simulink model "CMOS_Kernel_Memory_Sync"  (R2023b)
settings: Solver=VariableStepAuto  StartTime=0.0  StopTime=30000000  RelTol=1e-3
values from neighbouring files (symbols this model uses):
  AmountOfPixelsPerScanline = 400    [Kernel_Setup_Script.m]
  AmountOfRamBlocksScanlines = 5    [Kernel_Setup_Script.m]
  AmountOfRamBlocksScanlinesOffset = AmountOfRamBlocksScanlines - 1    (= 4)    [Kernel_Setup_Script.m]
  AmountOfScanlinePixels = 73700    [Kernel_Setup_Script.m]
  AmountOfScanlinePixelsOffset = AmountOfScanlinePixels - 1    (= 73699)    [Kernel_Setup_Script.m]
  AmountOfScanlines = 1100    [Kernel_Setup_Script.m]
  AmountOfScanlinesOffset = AmountOfScanlines - 1    (= 1099)    [Kernel_Setup_Script.m]
  AOPPK_Off = AmountOfPixelsPerScanline - 1    (= 399)    [Kernel_Setup_Script.m]
  AOPPS_Off = AmountOfPixelsPerScanline - 1    (= 399)    [Kernel_Setup_Script.m]
  FramePackOff_0 = FramePackOff_0 - ScanlineFifoCheck    [Kernel_Setup_Script.m]
  FramePackOff_1 = FramePackOff_1 - ScanlineFifoCheck    [Kernel_Setup_Script.m]
  FramePackOff_2 = FramePackOff_2 - ScanlineFifoCheck    [Kernel_Setup_Script.m]
  FramePackOff_3 = FramePackOff_3 - ScanlineFifoCheck    [Kernel_Setup_Script.m]
  FramePackOff_4 = FramePackOff_4 - ScanlineFifoCheck    [Kernel_Setup_Script.m]
  FramePackOff_5 = FramePackOff_5 - ScanlineFifoCheck    [Kernel_Setup_Script.m]
  KernelPackOff_0 = KernelPackOff_0 - KernelBitsPerRow    [Kernel_Setup_Script.m]
  KernelPackOff_1 = KernelPackOff_1 - KernelBitsPerRow    [Kernel_Setup_Script.m]
  KernelPackOff_2 = KernelPackOff_2 - KernelBitsPerRow    [Kernel_Setup_Script.m]
  KernelPackOff_3 = KernelPackOff_3 - KernelBitsPerRow    [Kernel_Setup_Script.m]
  Slice59DownTo48Top = (MsbOffset - (ScanlinePixelBitSizeController*1))    (= 59)    [Kernel_Setup_Script.m]
  Slice71DownTo60Top = (MsbOffset - (ScanlinePixelBitSizeController*0))    (= 71)    [Kernel_Setup_Script.m]
  TotalSectionsForFrames = AmountOfScanlines/AmountOfRamBlocksScanlines    (= 220)    [Kernel_Setup_Script.m]
  UltraRamRows = AmountOfPixelsPerScanline/ScanlineFifoCheck    [Kernel_Setup_Script.m]
  UltraRamRowsCeil = ceil(AmountOfPixelsPerScanline/ScanlineFifoCheck)    [Kernel_Setup_Script.m]
  UltraRamRowsKernel = AmountOfPixelsPerScanline/KernelBitsPerRow    (= 100)    [Kernel_Setup_Script.m]
  UltraRamRowsKernelCeil = ceil(AmountOfPixelsPerScanline/KernelBitsPerRow)    [Kernel_Setup_Script.m]
  UltraRamRowsMemorySectionOffset = UltraRamRowsCeil*AmountOfRamBlocksScanlines    [Kernel_Setup_Script.m]
  UltraRamRowsOffset = UltraRamRowsCeil - 1    [Kernel_Setup_Script.m]
undefined symbols (not defined in the file or in its folder): c, Down, sfvc784, Up, xck26
libraries: hdlBasic x4512, vmcUtilities x1
(part 35 of 39)

== system CMOS_Kernel_Memory_Sync/Memory Handler/Math/Kernel Result 9/Accumulator Offset 0 ==
  Input Value : Inport
  Input Valid : Inport  Port=2
  Last Row : Inport  Port=3
  Hard Reset : Inport  Port=4
  Accumulator 0 : hdlBasic/Accumulator  operation=Add  n_bits=64  overflow=Wrap  scale=1  rst=on  hasbypass=off  en=off  latency=1  msb_inp=100  msb=100  lsb=-100  use_behavioral_HDL=on  implementation=Fabric  XmcBlockStatus=1  maskContainerNames=group3  block_type=accum  block_config=sysgen:Accum_config  block_width=566  block_height=845
  Constant : hdlBasic/Constant  const=0  gui_display_data_type=Fixed-point  arith_type=Unsigned  n_bits=18  bin_pt=0  preci_type=Single  exp_width=8  frac_width=24  explicit_period=off  period=1  XmcBlockStatus=1  maskContainerNames=tabcontainer1  block_type=constant  block_config=sysgen:Constant_config
  Delay1 : hdlBasic/Delay  rst=off  en=off  latency=1  reg_retiming=off  XmcBlockStatus=1  maskContainerNames=group1  block_type=delay  block_config=sysgen:Delay_config
  Delay2 : hdlBasic/Delay  rst=off  en=off  latency=1  reg_retiming=off  XmcBlockStatus=1  maskContainerNames=group1  block_type=delay  block_config=sysgen:Delay_config
  Logical : hdlBasic/Logical  logical_function=AND  inputs=2  en=off  latency=1  precision=Full  arith_type=Unsigned  n_bits=16  bin_pt=0  align_bp=on  overflow=[]  quantization=[]  XmcBlockStatus=1  maskContainerNames=tabcontainer1  block_type=logical  block_config=sysgen:Logical_config
  Logical1 : hdlBasic/Logical  logical_function=OR  inputs=2  en=off  latency=1  precision=Full  arith_type=Unsigned  n_bits=16  bin_pt=0  align_bp=on  overflow=[]  quantization=[]  XmcBlockStatus=1  maskContainerNames=tabcontainer1  block_type=logical  block_config=sysgen:Logical_config
  Mux : hdlBasic/Mux  inputs=2  en=off  latency=1  precision=Full  arith_type=Unsigned  n_bits=16  bin_pt=14  quantization=Truncate  overflow=Wrap  XmcBlockStatus=1  maskContainerNames=tabcontainer1  block_type=mux  block_config=sysgen:Mux_config
  Accumulator Output : Outport
  Accumulator Valid : Outport  Port=2
  wires:
  Accumulator 0/1 -> Accumulator Output/1
  Input Valid/1 -> Logical/1, Mux/1
  Input Value/1 -> Mux/3
  Mux/1 -> Accumulator 0/1
  Last Row/1 -> Logical/2
  Constant/1 -> Mux/2
  Delay1/1 -> Accumulator 0/2
  Logical/1 -> Logical1/2, Delay2/1
  Delay2/1 -> Accumulator Valid/1
  Logical1/1 -> Delay1/1
  Hard Reset/1 -> Logical1/1

== system CMOS_Kernel_Memory_Sync/Memory Handler/Math/Kernel Result 9/Accumulator Offset 1 ==
  Input Value : Inport
  Input Valid : Inport  Port=2
  Last Row : Inport  Port=3
  Hard Reset : Inport  Port=4
  Accumulator 0 : hdlBasic/Accumulator  operation=Add  n_bits=64  overflow=Wrap  scale=1  rst=on  hasbypass=off  en=off  latency=1  msb_inp=100  msb=100  lsb=-100  use_behavioral_HDL=on  implementation=Fabric  XmcBlockStatus=1  maskContainerNames=group3  block_type=accum  block_config=sysgen:Accum_config  block_width=566  block_height=845
  Constant : hdlBasic/Constant  const=0  gui_display_data_type=Fixed-point  arith_type=Unsigned  n_bits=18  bin_pt=0  preci_type=Single  exp_width=8  frac_width=24  explicit_period=off  period=1  XmcBlockStatus=1  maskContainerNames=tabcontainer1  block_type=constant  block_config=sysgen:Constant_config
  Delay1 : hdlBasic/Delay  rst=off  en=off  latency=1  reg_retiming=off  XmcBlockStatus=1  maskContainerNames=group1  block_type=delay  block_config=sysgen:Delay_config
  Delay2 : hdlBasic/Delay  rst=off  en=off  latency=1  reg_retiming=off  XmcBlockStatus=1  maskContainerNames=group1  block_type=delay  block_config=sysgen:Delay_config
  Logical : hdlBasic/Logical  logical_function=AND  inputs=2  en=off  latency=1  precision=Full  arith_type=Unsigned  n_bits=16  bin_pt=0  align_bp=on  overflow=[]  quantization=[]  XmcBlockStatus=1  maskContainerNames=tabcontainer1  block_type=logical  block_config=sysgen:Logical_config
  Logical1 : hdlBasic/Logical  logical_function=OR  inputs=2  en=off  latency=1  precision=Full  arith_type=Unsigned  n_bits=16  bin_pt=0  align_bp=on  overflow=[]  quantization=[]  XmcBlockStatus=1  maskContainerNames=tabcontainer1  block_type=logical  block_config=sysgen:Logical_config
  Mux : hdlBasic/Mux  inputs=2  en=off  latency=1  precision=Full  arith_type=Unsigned  n_bits=16  bin_pt=14  quantization=Truncate  overflow=Wrap  XmcBlockStatus=1  maskContainerNames=tabcontainer1  block_type=mux  block_config=sysgen:Mux_config
  Accumulator Output : Outport
  Accumulator Valid : Outport  Port=2
  wires:
  Accumulator 0/1 -> Accumulator Output/1
  Input Valid/1 -> Logical/1, Mux/1
  Input Value/1 -> Mux/3
  Mux/1 -> Accumulator 0/1
  Last Row/1 -> Logical/2
  Constant/1 -> Mux/2
  Delay1/1 -> Accumulator 0/2
  Logical/1 -> Logical1/2, Delay2/1
  Delay2/1 -> Accumulator Valid/1
  Logical1/1 -> Delay1/1
  Hard Reset/1 -> Logical1/1

== system CMOS_Kernel_Memory_Sync/Memory Handler/Math/Kernel Result 9/Accumulator Offset 2 ==
  Input Value : Inport
  Input Valid : Inport  Port=2
  Last Row : Inport  Port=3
  Hard Reset : Inport  Port=4
  Accumulator 0 : hdlBasic/Accumulator  operation=Add  n_bits=64  overflow=Wrap  scale=1  rst=on  hasbypass=off  en=off  latency=1  msb_inp=100  msb=100  lsb=-100  use_behavioral_HDL=on  implementation=Fabric  XmcBlockStatus=1  maskContainerNames=group3  block_type=accum  block_config=sysgen:Accum_config  block_width=566  block_height=845
  Constant : hdlBasic/Constant  const=0  gui_display_data_type=Fixed-point  arith_type=Unsigned  n_bits=18  bin_pt=0  preci_type=Single  exp_width=8  frac_width=24  explicit_period=off  period=1  XmcBlockStatus=1  maskContainerNames=tabcontainer1  block_type=constant  block_config=sysgen:Constant_config
  Delay1 : hdlBasic/Delay  rst=off  en=off  latency=1  reg_retiming=off  XmcBlockStatus=1  maskContainerNames=group1  block_type=delay  block_config=sysgen:Delay_config
  Delay2 : hdlBasic/Delay  rst=off  en=off  latency=1  reg_retiming=off  XmcBlockStatus=1  maskContainerNames=group1  block_type=delay  block_config=sysgen:Delay_config
  Logical : hdlBasic/Logical  logical_function=AND  inputs=2  en=off  latency=1  precision=Full  arith_type=Unsigned  n_bits=16  bin_pt=0  align_bp=on  overflow=[]  quantization=[]  XmcBlockStatus=1  maskContainerNames=tabcontainer1  block_type=logical  block_config=sysgen:Logical_config
  Logical1 : hdlBasic/Logical  logical_function=OR  inputs=2  en=off  latency=1  precision=Full  arith_type=Unsigned  n_bits=16  bin_pt=0  align_bp=on  overflow=[]  quantization=[]  XmcBlockStatus=1  maskContainerNames=tabcontainer1  block_type=logical  block_config=sysgen:Logical_config
  Mux : hdlBasic/Mux  inputs=2  en=off  latency=1  precision=Full  arith_type=Unsigned  n_bits=16  bin_pt=14  quantization=Truncate  overflow=Wrap  XmcBlockStatus=1  maskContainerNames=tabcontainer1  block_type=mux  block_config=sysgen:Mux_config
  Accumulator Output : Outport
  Accumulator Valid : Outport  Port=2
  wires:
  Accumulator 0/1 -> Accumulator Output/1
  Input Valid/1 -> Logical/1, Mux/1
  Input Value/1 -> Mux/3
  Mux/1 -> Accumulator 0/1
  Last Row/1 -> Logical/2
  Constant/1 -> Mux/2
  Delay1/1 -> Accumulator 0/2
  Logical/1 -> Logical1/2, Delay2/1
  Delay2/1 -> Accumulator Valid/1
  Logical1/1 -> Delay1/1
  Hard Reset/1 -> Logical1/1

== system CMOS_Kernel_Memory_Sync/Memory Handler/Math/Kernel Result 9/Accumulator Offset 3 ==
  Input Value : Inport
  Input Valid : Inport  Port=2
  Last Row : Inport  Port=3
  Hard Reset : Inport  Port=4
  Accumulator 0 : hdlBasic/Accumulator  operation=Add  n_bits=64  overflow=Wrap  scale=1  rst=on  hasbypass=off  en=off  latency=1  msb_inp=100  msb=100  lsb=-100  use_behavioral_HDL=on  implementation=Fabric  XmcBlockStatus=1  maskContainerNames=group3  block_type=accum  block_config=sysgen:Accum_config  block_width=566  block_height=845
  Constant : hdlBasic/Constant  const=0  gui_display_data_type=Fixed-point  arith_type=Unsigned  n_bits=18  bin_pt=0  preci_type=Single  exp_width=8  frac_width=24  explicit_period=off  period=1  XmcBlockStatus=1  maskContainerNames=tabcontainer1  block_type=constant  block_config=sysgen:Constant_config
  Delay1 : hdlBasic/Delay  rst=off  en=off  latency=1  reg_retiming=off  XmcBlockStatus=1  maskContainerNames=group1  block_type=delay  block_config=sysgen:Delay_config
  Delay2 : hdlBasic/Delay  rst=off  en=off  latency=1  reg_retiming=off  XmcBlockStatus=1  maskContainerNames=group1  block_type=delay  block_config=sysgen:Delay_config
  Logical : hdlBasic/Logical  logical_function=AND  inputs=2  en=off  latency=1  precision=Full  arith_type=Unsigned  n_bits=16  bin_pt=0  align_bp=on  overflow=[]  quantization=[]  XmcBlockStatus=1  maskContainerNames=tabcontainer1  block_type=logical  block_config=sysgen:Logical_config
  Logical1 : hdlBasic/Logical  logical_function=OR  inputs=2  en=off  latency=1  precision=Full  arith_type=Unsigned  n_bits=16  bin_pt=0  align_bp=on  overflow=[]  quantization=[]  XmcBlockStatus=1  maskContainerNames=tabcontainer1  block_type=logical  block_config=sysgen:Logical_config
  Mux : hdlBasic/Mux  inputs=2  en=off  latency=1  precision=Full  arith_type=Unsigned  n_bits=16  bin_pt=14  quantization=Truncate  overflow=Wrap  XmcBlockStatus=1  maskContainerNames=tabcontainer1  block_type=mux  block_config=sysgen:Mux_config
  Accumulator Output : Outport
  Accumulator Valid : Outport  Port=2
  wires:
  Accumulator 0/1 -> Accumulator Output/1
  Input Valid/1 -> Logical/1, Mux/1
  Input Value/1 -> Mux/3
  Mux/1 -> Accumulator 0/1
  Last Row/1 -> Logical/2
  Constant/1 -> Mux/2
  Delay1/1 -> Accumulator 0/2
  Logical/1 -> Logical1/2, Delay2/1
  Delay2/1 -> Accumulator Valid/1
  Logical1/1 -> Delay1/1
  Hard Reset/1 -> Logical1/1

== system CMOS_Kernel_Memory_Sync/Memory Handler/Math/Kernel Result 9/Accumulator Offset 4 ==
  Input Value : Inport
  Input Valid : Inport  Port=2
  Last Row : Inport  Port=3
  Hard Reset : Inport  Port=4
  Accumulator 0 : hdlBasic/Accumulator  operation=Add  n_bits=64  overflow=Wrap  scale=1  rst=on  hasbypass=off  en=off  latency=1  msb_inp=100  msb=100  lsb=-100  use_behavioral_HDL=on  implementation=Fabric  XmcBlockStatus=1  maskContainerNames=group3  block_type=accum  block_config=sysgen:Accum_config  block_width=566  block_height=845
  Constant : hdlBasic/Constant  const=0  gui_display_data_type=Fixed-point  arith_type=Unsigned  n_bits=18  bin_pt=0  preci_type=Single  exp_width=8  frac_width=24  explicit_period=off  period=1  XmcBlockStatus=1  maskContainerNames=tabcontainer1  block_type=constant  block_config=sysgen:Constant_config
  Delay1 : hdlBasic/Delay  rst=off  en=off  latency=1  reg_retiming=off  XmcBlockStatus=1  maskContainerNames=group1  block_type=delay  block_config=sysgen:Delay_config
  Delay2 : hdlBasic/Delay  rst=off  en=off  latency=1  reg_retiming=off  XmcBlockStatus=1  maskContainerNames=group1  block_type=delay  block_config=sysgen:Delay_config
  Logical : hdlBasic/Logical  logical_function=AND  inputs=2  en=off  latency=1  precision=Full  arith_type=Unsigned  n_bits=16  bin_pt=0  align_bp=on  overflow=[]  quantization=[]  XmcBlockStatus=1  maskContainerNames=tabcontainer1  block_type=logical  block_config=sysgen:Logical_config
  Logical1 : hdlBasic/Logical  logical_function=OR  inputs=2  en=off  latency=1  precision=Full  arith_type=Unsigned  n_bits=16  bin_pt=0  align_bp=on  overflow=[]  quantization=[]  XmcBlockStatus=1  maskContainerNames=tabcontainer1  block_type=logical  block_config=sysgen:Logical_config
  Mux : hdlBasic/Mux  inputs=2  en=off  latency=1  precision=Full  arith_type=Unsigned  n_bits=16  bin_pt=14  quantization=Truncate  overflow=Wrap  XmcBlockStatus=1  maskContainerNames=tabcontainer1  block_type=mux  block_config=sysgen:Mux_config
  Accumulator Output : Outport
  Accumulator Valid : Outport  Port=2
  wires:
  Accumulator 0/1 -> Accumulator Output/1
  Input Valid/1 -> Logical/1, Mux/1
  Input Value/1 -> Mux/3
  Mux/1 -> Accumulator 0/1
  Last Row/1 -> Logical/2
  Constant/1 -> Mux/2
  Delay1/1 -> Accumulator 0/2
  Logical/1 -> Logical1/2, Delay2/1
  Delay2/1 -> Accumulator Valid/1
  Logical1/1 -> Delay1/1
  Hard Reset/1 -> Logical1/1

== system CMOS_Kernel_Memory_Sync/Memory Handler/Math/Kernel Result 9/Multiple and Add Offset 0 ==
  Pixel 0 : Inport
  Weight 0 : Inport  Port=2
  Pixel 1 : Inport  Port=3
  Weight 1 : Inport  Port=4
  Pixel 2 : Inport  Port=5
  Weight 2 : Inport  Port=6
  Pixel 3 : Inport  Port=7
  Weight 3 : Inport  Port=8
  Pixel 4 : Inport  Port=9
  Weight 4 : Inport  Port=10
  Pixel 5 : Inport  Port=11
  Weight 5 : Inport  Port=12
  Pixel 6 : Inport  Port=13
  Weight 6 : Inport  Port=14
  Pixel 7 : Inport  Port=15
  Weight 7 : Inport  Port=16
  Pixel 8 : Inport  Port=17
  Weight 8 : Inport  Port=18
  Pixel 9 : Inport  Port=19
  Weight 9 : Inport  Port=20
  Pixel 10 : Inport  Port=21
  Weight 10 : Inport  Port=22
  Pixel 11 : Inport  Port=23
  Weight 11 : Inport  Port=24
  Valid Data : Inport  Port=25
  "Combine ((0-1)-(2-3)) - ((4-5)-(6-7)) " : hdlBasic/AddSub  mode=Addition  use_carryin=off  use_carryout=off  en=off  latency=1  precision=Full  arith_type=Unsigned  n_bits=21  bin_pt=0  quantization=Truncate  overflow=Wrap  use_behavioral_HDL=off  hw_selection=Fabric  pipelined=off  XmcBlockStatus=1  maskContainerNames=tabcontainer1  block_type=addsub  block_config=sysgen:Addsub_config
  Combine (0-1)-(2-3) : hdlBasic/AddSub  mode=Addition  use_carryin=off  use_carryout=off  en=off  latency=1  precision=Full  arith_type=Unsigned  n_bits=20  bin_pt=0  quantization=Truncate  overflow=Wrap  use_behavioral_HDL=off  hw_selection=Fabric  pipelined=off  XmcBlockStatus=1  maskContainerNames=tabcontainer1  block_type=addsub  block_config=sysgen:Addsub_config
  Combine (4-5)-(6-7) : hdlBasic/AddSub  mode=Addition  use_carryin=off  use_carryout=off  en=off  latency=1  precision=Full  arith_type=Unsigned  n_bits=20  bin_pt=0  quantization=Truncate  overflow=Wrap  use_behavioral_HDL=off  hw_selection=Fabric  pipelined=off  XmcBlockStatus=1  maskContainerNames=tabcontainer1  block_type=addsub  block_config=sysgen:Addsub_config
  Combine (8-9)-(10-11) : hdlBasic/AddSub  mode=Addition  use_carryin=off  use_carryout=off  en=off  latency=1  precision=Full  arith_type=Unsigned  n_bits=20  bin_pt=0  quantization=Truncate  overflow=Wrap  use_behavioral_HDL=off  hw_selection=Fabric  pipelined=off  XmcBlockStatus=1  maskContainerNames=tabcontainer1  block_type=addsub  block_config=sysgen:Addsub_config
  Combine 0-1 : hdlBasic/AddSub  mode=Addition  use_carryin=off  use_carryout=off  en=off  latency=1  precision=Full  arith_type=Unsigned  n_bits=31  bin_pt=0  quantization=Truncate  overflow=Wrap  use_behavioral_HDL=off  hw_selection=Fabric  pipelined=off  XmcBlockStatus=1  maskContainerNames=tabcontainer1  block_type=addsub  block_config=sysgen:Addsub_config
  Combine 10-11 : hdlBasic/AddSub  mode=Addition  use_carryin=off  use_carryout=off  en=off  latency=1  precision=Full  arith_type=Unsigned  n_bits=19  bin_pt=0  quantization=Truncate  overflow=Wrap  use_behavioral_HDL=off  hw_selection=Fabric  pipelined=off  XmcBlockStatus=1  maskContainerNames=tabcontainer1  block_type=addsub  block_config=sysgen:Addsub_config
  Combine 2-3 : hdlBasic/AddSub  mode=Addition  use_carryin=off  use_carryout=off  en=off  latency=1  precision=Full  arith_type=Unsigned  n_bits=19  bin_pt=0  quantization=Truncate  overflow=Wrap  use_behavioral_HDL=off  hw_selection=Fabric  pipelined=off  XmcBlockStatus=1  maskContainerNames=tabcontainer1  block_type=addsub  block_config=sysgen:Addsub_config
  Combine 4-5 : hdlBasic/AddSub  mode=Addition  use_carryin=off  use_carryout=off  en=off  latency=1  precision=Full  arith_type=Unsigned  n_bits=19  bin_pt=0  quantization=Truncate  overflow=Wrap  use_behavioral_HDL=off  hw_selection=Fabric  pipelined=off  XmcBlockStatus=1  maskContainerNames=tabcontainer1  block_type=addsub  block_config=sysgen:Addsub_config
  Combine 6-7 : hdlBasic/AddSub  mode=Addition  use_carryin=off  use_carryout=off  en=off  latency=1  precision=Full  arith_type=Unsigned  n_bits=19  bin_pt=0  quantization=Truncate  overflow=Wrap  use_behavioral_HDL=off  hw_selection=Fabric  pipelined=off  XmcBlockStatus=1  maskContainerNames=tabcontainer1  block_type=addsub  block_config=sysgen:Addsub_config
  Combine 8-9 : hdlBasic/AddSub  mode=Addition  use_carryin=off  use_carryout=off  en=off  latency=1  precision=Full  arith_type=Unsigned  n_bits=19  bin_pt=0  quantization=Truncate  overflow=Wrap  use_behavioral_HDL=off  hw_selection=Fabric  pipelined=off  XmcBlockStatus=1  maskContainerNames=tabcontainer1  block_type=addsub  block_config=sysgen:Addsub_config
  Delay Addition{,2..4} (4 alike) : hdlBasic/Delay  rst=off  en=off  latency=1  reg_retiming=off  XmcBlockStatus=1  maskContainerNames=group1  block_type=delay  block_config=sysgen:Delay_config
  Delay Addition 2 : hdlBasic/Delay  rst=off  en=off  latency=1  reg_retiming=off  XmcBlockStatus=1  maskContainerNames=group1  block_type=delay  block_config=sysgen:Delay_config
  Delay Addition1 : hdlBasic/Delay  rst=off  en=off  latency=3  reg_retiming=off  XmcBlockStatus=1  maskContainerNames=group1  block_type=delay  block_config=sysgen:Delay_config
  Last Combine : hdlBasic/AddSub  mode=Addition  use_carryin=off  use_carryout=off  en=off  latency=1  precision=Full  arith_type=Unsigned  n_bits=22  bin_pt=0  quantization=Truncate  overflow=Wrap  use_behavioral_HDL=off  hw_selection=Fabric  pipelined=off  XmcBlockStatus=1  maskContainerNames=tabcontainer1  block_type=addsub  block_config=sysgen:Addsub_config
  Pixel 0 X Weight 0 : hdlBasic/Mult  precision=User Defined  arith_type=Unsigned  n_bits=30  bin_pt=0  quantization=Truncate  overflow=Wrap  en=off  latency=3  use_behavioral_HDL=off  opt=Speed  use_embedded=on  optimum_pipeline=off  pipeline=on  use_rpm=on  placement_style=Triangular  XmcBlockStatus=1  maskContainerNames=group1  block_type=mult  block_config=sysgen:Mult_config  block_width=598  block_height=876
  Pixel 1 X Weight 1 : hdlBasic/Mult  precision=User Defined  arith_type=Unsigned  n_bits=30  bin_pt=0  quantization=Truncate  overflow=Wrap  en=off  latency=3  use_behavioral_HDL=off  opt=Speed  use_embedded=on  optimum_pipeline=off  pipeline=on  use_rpm=on  placement_style=Triangular  XmcBlockStatus=1  maskContainerNames=group1  block_type=mult  block_config=sysgen:Mult_config  block_width=598  block_height=876
  Pixel 10 X Weight 10 : hdlBasic/Mult  precision=User Defined  arith_type=Unsigned  n_bits=30  bin_pt=0  quantization=Truncate  overflow=Wrap  en=off  latency=3  use_behavioral_HDL=off  opt=Speed  use_embedded=on  optimum_pipeline=off  pipeline=on  use_rpm=on  placement_style=Triangular  XmcBlockStatus=1  maskContainerNames=group1  block_type=mult  block_config=sysgen:Mult_config  block_width=598  block_height=876
  Pixel 11 X Weight 11 : hdlBasic/Mult  precision=User Defined  arith_type=Unsigned  n_bits=30  bin_pt=0  quantization=Truncate  overflow=Wrap  en=off  latency=3  use_behavioral_HDL=off  opt=Speed  use_embedded=on  optimum_pipeline=off  pipeline=on  use_rpm=on  placement_style=Triangular  XmcBlockStatus=1  maskContainerNames=group1  block_type=mult  block_config=sysgen:Mult_config  block_width=598  block_height=876
  Pixel 2 X Weight 2 : hdlBasic/Mult  precision=User Defined  arith_type=Unsigned  n_bits=30  bin_pt=0  quantization=Truncate  overflow=Wrap  en=off  latency=3  use_behavioral_HDL=off  opt=Speed  use_embedded=on  optimum_pipeline=off  pipeline=on  use_rpm=on  placement_style=Triangular  XmcBlockStatus=1  maskContainerNames=group1  block_type=mult  block_config=sysgen:Mult_config  block_width=598  block_height=876
  Pixel 3 X Weight 3 : hdlBasic/Mult  precision=User Defined  arith_type=Unsigned  n_bits=30  bin_pt=0  quantization=Truncate  overflow=Wrap  en=off  latency=3  use_behavioral_HDL=off  opt=Speed  use_embedded=on  optimum_pipeline=off  pipeline=on  use_rpm=on  placement_style=Triangular  XmcBlockStatus=1  maskContainerNames=group1  block_type=mult  block_config=sysgen:Mult_config  block_width=598  block_height=876
  Pixel 4 X Weight 4 : hdlBasic/Mult  precision=User Defined  arith_type=Unsigned  n_bits=30  bin_pt=0  quantization=Truncate  overflow=Wrap  en=off  latency=3  use_behavioral_HDL=off  opt=Speed  use_embedded=on  optimum_pipeline=off  pipeline=on  use_rpm=on  placement_style=Triangular  XmcBlockStatus=1  maskContainerNames=group1  block_type=mult  block_config=sysgen:Mult_config  block_width=598  block_height=876
  Pixel 5 X Weight 5 : hdlBasic/Mult  precision=User Defined  arith_type=Unsigned  n_bits=30  bin_pt=0  quantization=Truncate  overflow=Wrap  en=off  latency=3  use_behavioral_HDL=off  opt=Speed  use_embedded=on  optimum_pipeline=off  pipeline=on  use_rpm=on  placement_style=Triangular  XmcBlockStatus=1  maskContainerNames=group1  block_type=mult  block_config=sysgen:Mult_config  block_width=598  block_height=876
  Pixel 6 X Weight 6 : hdlBasic/Mult  precision=User Defined  arith_type=Unsigned  n_bits=30  bin_pt=0  quantization=Truncate  overflow=Wrap  en=off  latency=3  use_behavioral_HDL=off  opt=Speed  use_embedded=on  optimum_pipeline=off  pipeline=on  use_rpm=on  placement_style=Triangular  XmcBlockStatus=1  maskContainerNames=group1  block_type=mult  block_config=sysgen:Mult_config  block_width=598  block_height=876
  Pixel 7 X Weight 7 : hdlBasic/Mult  precision=User Defined  arith_type=Unsigned  n_bits=30  bin_pt=0  quantization=Truncate  overflow=Wrap  en=off  latency=3  use_behavioral_HDL=off  opt=Speed  use_embedded=on  optimum_pipeline=off  pipeline=on  use_rpm=on  placement_style=Triangular  XmcBlockStatus=1  maskContainerNames=group1  block_type=mult  block_config=sysgen:Mult_config  block_width=598  block_height=876
  Pixel 8 X Weight 8 : hdlBasic/Mult  precision=User Defined  arith_type=Unsigned  n_bits=30  bin_pt=0  quantization=Truncate  overflow=Wrap  en=off  latency=3  use_behavioral_HDL=off  opt=Speed  use_embedded=on  optimum_pipeline=off  pipeline=on  use_rpm=on  placement_style=Triangular  XmcBlockStatus=1  maskContainerNames=group1  block_type=mult  block_config=sysgen:Mult_config  block_width=598  block_height=876
  Pixel 9 X Weight 9 : hdlBasic/Mult  precision=User Defined  arith_type=Unsigned  n_bits=30  bin_pt=0  quantization=Truncate  overflow=Wrap  en=off  latency=3  use_behavioral_HDL=off  opt=Speed  use_embedded=on  optimum_pipeline=off  pipeline=on  use_rpm=on  placement_style=Triangular  XmcBlockStatus=1  maskContainerNames=group1  block_type=mult  block_config=sysgen:Mult_config  block_width=598  block_height=876
  Slice Out : Outport
  Valid Out : Outport  Port=2
  wires:
  Pixel 9 X Weight 9/1 -> Combine 8-9/2
  Pixel 7 X Weight 7/1 -> Combine 6-7/2
  Combine (8-9)-(10-11)/1 -> Delay Addition/1
  Combine 10-11/1 -> Combine (8-9)-(10-11)/2
  Pixel 8 X Weight 8/1 -> Combine 8-9/1
  Pixel 10 X Weight 10/1 -> Combine 10-11/1
  Combine (0-1)-(2-3)/1 -> "Combine ((0-1)-(2-3)) - ((4-5)-(6-7)) "/1
  Pixel 1 X Weight 1/1 -> Combine 0-1/2
  Pixel 6 X Weight 6/1 -> Combine 6-7/1
  Combine 6-7/1 -> Combine (4-5)-(6-7)/2
  Combine 4-5/1 -> Combine (4-5)-(6-7)/1
  Combine (4-5)-(6-7)/1 -> "Combine ((0-1)-(2-3)) - ((4-5)-(6-7)) "/2
  Pixel 2 X Weight 2/1 -> Combine 2-3/1
  Pixel 4 X Weight 4/1 -> Combine 4-5/1
  Combine 0-1/1 -> Combine (0-1)-(2-3)/1
  Pixel 5 X Weight 5/1 -> Combine 4-5/2
  Pixel 0 X Weight 0/1 -> Combine 0-1/1
  Pixel 3 X Weight 3/1 -> Combine 2-3/2
  Combine 8-9/1 -> Combine (8-9)-(10-11)/1
  Pixel 11 X Weight 11/1 -> Combine 10-11/2
  Combine 2-3/1 -> Combine (0-1)-(2-3)/2
  Last Combine/1 -> Slice Out/1
  "Combine ((0-1)-(2-3)) - ((4-5)-(6-7)) "/1 -> Last Combine/1
  Delay Addition/1 -> Last Combine/2
  Pixel 0/1 -> Pixel 0 X Weight 0/1
  Weight 0/1 -> Pixel 0 X Weight 0/2
  Pixel 1/1 -> Pixel 1 X Weight 1/1
  Weight 1/1 -> Pixel 1 X Weight 1/2
  Pixel 2/1 -> Pixel 2 X Weight 2/1
  Weight 2/1 -> Pixel 2 X Weight 2/2
  Pixel 3/1 -> Pixel 3 X Weight 3/1
  Weight 3/1 -> Pixel 3 X Weight 3/2
  Pixel 4/1 -> Pixel 4 X Weight 4/1
  Weight 4/1 -> Pixel 4 X Weight 4/2
  Pixel 5/1 -> Pixel 5 X Weight 5/1
  Weight 5/1 -> Pixel 5 X Weight 5/2
  Pixel 6/1 -> Pixel 6 X Weight 6/1
  Weight 6/1 -> Pixel 6 X Weight 6/2
  Pixel 7/1 -> Pixel 7 X Weight 7/1
  Weight 7/1 -> Pixel 7 X Weight 7/2
  Pixel 8/1 -> Pixel 8 X Weight 8/1
  Weight 8/1 -> Pixel 8 X Weight 8/2
  Pixel 9/1 -> Pixel 9 X Weight 9/1
  Weight 9/1 -> Pixel 9 X Weight 9/2
  Pixel 10/1 -> Pixel 10 X Weight 10/1
  Weight 10/1 -> Pixel 10 X Weight 10/2
  Pixel 11/1 -> Pixel 11 X Weight 11/1
  Weight 11/1 -> Pixel 11 X Weight 11/2
  Valid Data/1 -> Delay Addition1/1
  Delay Addition1/1 -> Delay Addition 2/1
  Delay Addition 2/1 -> Delay Addition2/1
  Delay Addition2/1 -> Delay Addition3/1
  Delay Addition3/1 -> Delay Addition4/1
  Delay Addition4/1 -> Valid Out/1

== system CMOS_Kernel_Memory_Sync/Memory Handler/Math/Kernel Result 9/Multiple and Add Offset 1 ==
  Pixel 0 : Inport
  Weight 0 : Inport  Port=2
  Pixel 1 : Inport  Port=3
  Weight 1 : Inport  Port=4
  Pixel 2 : Inport  Port=5
  Weight 2 : Inport  Port=6
  Pixel 3 : Inport  Port=7
  Weight 3 : Inport  Port=8
  Pixel 4 : Inport  Port=9
  Weight 4 : Inport  Port=10
  Pixel 5 : Inport  Port=11
  Weight 5 : Inport  Port=12
  Pixel 6 : Inport  Port=13
  Weight 6 : Inport  Port=14
  Pixel 7 : Inport  Port=15
  Weight 7 : Inport  Port=16
  Pixel 8 : Inport  Port=17
  Weight 8 : Inport  Port=18
  Pixel 9 : Inport  Port=19
  Weight 9 : Inport  Port=20
  Pixel 10 : Inport  Port=21
  Weight 10 : Inport  Port=22
  Pixel 11 : Inport  Port=23
  Weight 11 : Inport  Port=24
  Valid Data : Inport  Port=25
  "Combine ((0-1)-(2-3)) - ((4-5)-(6-7)) " : hdlBasic/AddSub  mode=Addition  use_carryin=off  use_carryout=off  en=off  latency=1  precision=Full  arith_type=Unsigned  n_bits=21  bin_pt=0  quantization=Truncate  overflow=Wrap  use_behavioral_HDL=off  hw_selection=Fabric  pipelined=off  XmcBlockStatus=1  maskContainerNames=tabcontainer1  block_type=addsub  block_config=sysgen:Addsub_config
  Combine (0-1)-(2-3) : hdlBasic/AddSub  mode=Addition  use_carryin=off  use_carryout=off  en=off  latency=1  precision=Full  arith_type=Unsigned  n_bits=20  bin_pt=0  quantization=Truncate  overflow=Wrap  use_behavioral_HDL=off  hw_selection=Fabric  pipelined=off  XmcBlockStatus=1  maskContainerNames=tabcontainer1  block_type=addsub  block_config=sysgen:Addsub_config
  Combine (4-5)-(6-7) : hdlBasic/AddSub  mode=Addition  use_carryin=off  use_carryout=off  en=off  latency=1  precision=Full  arith_type=Unsigned  n_bits=20  bin_pt=0  quantization=Truncate  overflow=Wrap  use_behavioral_HDL=off  hw_selection=Fabric  pipelined=off  XmcBlockStatus=1  maskContainerNames=tabcontainer1  block_type=addsub  block_config=sysgen:Addsub_config
  Combine (8-9)-(10-11) : hdlBasic/AddSub  mode=Addition  use_carryin=off  use_carryout=off  en=off  latency=1  precision=Full  arith_type=Unsigned  n_bits=20  bin_pt=0  quantization=Truncate  overflow=Wrap  use_behavioral_HDL=off  hw_selection=Fabric  pipelined=off  XmcBlockStatus=1  maskContainerNames=tabcontainer1  block_type=addsub  block_config=sysgen:Addsub_config
  Combine 0-1 : hdlBasic/AddSub  mode=Addition  use_carryin=off  use_carryout=off  en=off  latency=1  precision=Full  arith_type=Unsigned  n_bits=31  bin_pt=0  quantization=Truncate  overflow=Wrap  use_behavioral_HDL=off  hw_selection=Fabric  pipelined=off  XmcBlockStatus=1  maskContainerNames=tabcontainer1  block_type=addsub  block_config=sysgen:Addsub_config
  Combine 10-11 : hdlBasic/AddSub  mode=Addition  use_carryin=off  use_carryout=off  en=off  latency=1  precision=Full  arith_type=Unsigned  n_bits=19  bin_pt=0  quantization=Truncate  overflow=Wrap  use_behavioral_HDL=off  hw_selection=Fabric  pipelined=off  XmcBlockStatus=1  maskContainerNames=tabcontainer1  block_type=addsub  block_config=sysgen:Addsub_config
  Combine 2-3 : hdlBasic/AddSub  mode=Addition  use_carryin=off  use_carryout=off  en=off  latency=1  precision=Full  arith_type=Unsigned  n_bits=19  bin_pt=0  quantization=Truncate  overflow=Wrap  use_behavioral_HDL=off  hw_selection=Fabric  pipelined=off  XmcBlockStatus=1  maskContainerNames=tabcontainer1  block_type=addsub  block_config=sysgen:Addsub_config
  Combine 4-5 : hdlBasic/AddSub  mode=Addition  use_carryin=off  use_carryout=off  en=off  latency=1  precision=Full  arith_type=Unsigned  n_bits=19  bin_pt=0  quantization=Truncate  overflow=Wrap  use_behavioral_HDL=off  hw_selection=Fabric  pipelined=off  XmcBlockStatus=1  maskContainerNames=tabcontainer1  block_type=addsub  block_config=sysgen:Addsub_config
  Combine 6-7 : hdlBasic/AddSub  mode=Addition  use_carryin=off  use_carryout=off  en=off  latency=1  precision=Full  arith_type=Unsigned  n_bits=19  bin_pt=0  quantization=Truncate  overflow=Wrap  use_behavioral_HDL=off  hw_selection=Fabric  pipelined=off  XmcBlockStatus=1  maskContainerNames=tabcontainer1  block_type=addsub  block_config=sysgen:Addsub_config
  Combine 8-9 : hdlBasic/AddSub  mode=Addition  use_carryin=off  use_carryout=off  en=off  latency=1  precision=Full  arith_type=Unsigned  n_bits=19  bin_pt=0  quantization=Truncate  overflow=Wrap  use_behavioral_HDL=off  hw_selection=Fabric  pipelined=off  XmcBlockStatus=1  maskContainerNames=tabcontainer1  block_type=addsub  block_config=sysgen:Addsub_config
  Delay Addition{,2..4} (4 alike) : hdlBasic/Delay  rst=off  en=off  latency=1  reg_retiming=off  XmcBlockStatus=1  maskContainerNames=group1  block_type=delay  block_config=sysgen:Delay_config
  Delay Addition 2 : hdlBasic/Delay  rst=off  en=off  latency=1  reg_retiming=off  XmcBlockStatus=1  maskContainerNames=group1  block_type=delay  block_config=sysgen:Delay_config
  Delay Addition1 : hdlBasic/Delay  rst=off  en=off  latency=3  reg_retiming=off  XmcBlockStatus=1  maskContainerNames=group1  block_type=delay  block_config=sysgen:Delay_config
  Last Combine : hdlBasic/AddSub  mode=Addition  use_carryin=off  use_carryout=off  en=off  latency=1  precision=Full  arith_type=Unsigned  n_bits=22  bin_pt=0  quantization=Truncate  overflow=Wrap  use_behavioral_HDL=off  hw_selection=Fabric  pipelined=off  XmcBlockStatus=1  maskContainerNames=tabcontainer1  block_type=addsub  block_config=sysgen:Addsub_config
  Pixel 0 X Weight 0 : hdlBasic/Mult  precision=User Defined  arith_type=Unsigned  n_bits=30  bin_pt=0  quantization=Truncate  overflow=Wrap  en=off  latency=3  use_behavioral_HDL=off  opt=Speed  use_embedded=on  optimum_pipeline=off  pipeline=on  use_rpm=on  placement_style=Triangular  XmcBlockStatus=1  maskContainerNames=group1  block_type=mult  block_config=sysgen:Mult_config  block_width=598  block_height=876
  Pixel 1 X Weight 1 : hdlBasic/Mult  precision=User Defined  arith_type=Unsigned  n_bits=30  bin_pt=0  quantization=Truncate  overflow=Wrap  en=off  latency=3  use_behavioral_HDL=off  opt=Speed  use_embedded=on  optimum_pipeline=off  pipeline=on  use_rpm=on  placement_style=Triangular  XmcBlockStatus=1  maskContainerNames=group1  block_type=mult  block_config=sysgen:Mult_config  block_width=598  block_height=876
  Pixel 10 X Weight 10 : hdlBasic/Mult  precision=User Defined  arith_type=Unsigned  n_bits=30  bin_pt=0  quantization=Truncate  overflow=Wrap  en=off  latency=3  use_behavioral_HDL=off  opt=Speed  use_embedded=on  optimum_pipeline=off  pipeline=on  use_rpm=on  placement_style=Triangular  XmcBlockStatus=1  maskContainerNames=group1  block_type=mult  block_config=sysgen:Mult_config  block_width=598  block_height=876
  Pixel 11 X Weight 11 : hdlBasic/Mult  precision=User Defined  arith_type=Unsigned  n_bits=30  bin_pt=0  quantization=Truncate  overflow=Wrap  en=off  latency=3  use_behavioral_HDL=off  opt=Speed  use_embedded=on  optimum_pipeline=off  pipeline=on  use_rpm=on  placement_style=Triangular  XmcBlockStatus=1  maskContainerNames=group1  block_type=mult  block_config=sysgen:Mult_config  block_width=598  block_height=876
  Pixel 2 X Weight 2 : hdlBasic/Mult  precision=User Defined  arith_type=Unsigned  n_bits=30  bin_pt=0  quantization=Truncate  overflow=Wrap  en=off  latency=3  use_behavioral_HDL=off  opt=Speed  use_embedded=on  optimum_pipeline=off  pipeline=on  use_rpm=on  placement_style=Triangular  XmcBlockStatus=1  maskContainerNames=group1  block_type=mult  block_config=sysgen:Mult_config  block_width=598  block_height=876
  Pixel 3 X Weight 3 : hdlBasic/Mult  precision=User Defined  arith_type=Unsigned  n_bits=30  bin_pt=0  quantization=Truncate  overflow=Wrap  en=off  latency=3  use_behavioral_HDL=off  opt=Speed  use_embedded=on  optimum_pipeline=off  pipeline=on  use_rpm=on  placement_style=Triangular  XmcBlockStatus=1  maskContainerNames=group1  block_type=mult  block_config=sysgen:Mult_config  block_width=598  block_height=876
  Pixel 4 X Weight 4 : hdlBasic/Mult  precision=User Defined  arith_type=Unsigned  n_bits=30  bin_pt=0  quantization=Truncate  overflow=Wrap  en=off  latency=3  use_behavioral_HDL=off  opt=Speed  use_embedded=on  optimum_pipeline=off  pipeline=on  use_rpm=on  placement_style=Triangular  XmcBlockStatus=1  maskContainerNames=group1  block_type=mult  block_config=sysgen:Mult_config  block_width=598  block_height=876
  Pixel 5 X Weight 5 : hdlBasic/Mult  precision=User Defined  arith_type=Unsigned  n_bits=30  bin_pt=0  quantization=Truncate  overflow=Wrap  en=off  latency=3  use_behavioral_HDL=off  opt=Speed  use_embedded=on  optimum_pipeline=off  pipeline=on  use_rpm=on  placement_style=Triangular  XmcBlockStatus=1  maskContainerNames=group1  block_type=mult  block_config=sysgen:Mult_config  block_width=598  block_height=876
  Pixel 6 X Weight 6 : hdlBasic/Mult  precision=User Defined  arith_type=Unsigned  n_bits=30  bin_pt=0  quantization=Truncate  overflow=Wrap  en=off  latency=3  use_behavioral_HDL=off  opt=Speed  use_embedded=on  optimum_pipeline=off  pipeline=on  use_rpm=on  placement_style=Triangular  XmcBlockStatus=1  maskContainerNames=group1  block_type=mult  block_config=sysgen:Mult_config  block_width=598  block_height=876
  Pixel 7 X Weight 7 : hdlBasic/Mult  precision=User Defined  arith_type=Unsigned  n_bits=30  bin_pt=0  quantization=Truncate  overflow=Wrap  en=off  latency=3  use_behavioral_HDL=off  opt=Speed  use_embedded=on  optimum_pipeline=off  pipeline=on  use_rpm=on  placement_style=Triangular  XmcBlockStatus=1  maskContainerNames=group1  block_type=mult  block_config=sysgen:Mult_config  block_width=598  block_height=876
  Pixel 8 X Weight 8 : hdlBasic/Mult  precision=User Defined  arith_type=Unsigned  n_bits=30  bin_pt=0  quantization=Truncate  overflow=Wrap  en=off  latency=3  use_behavioral_HDL=off  opt=Speed  use_embedded=on  optimum_pipeline=off  pipeline=on  use_rpm=on  placement_style=Triangular  XmcBlockStatus=1  maskContainerNames=group1  block_type=mult  block_config=sysgen:Mult_config  block_width=598  block_height=876
  Pixel 9 X Weight 9 : hdlBasic/Mult  precision=User Defined  arith_type=Unsigned  n_bits=30  bin_pt=0  quantization=Truncate  overflow=Wrap  en=off  latency=3  use_behavioral_HDL=off  opt=Speed  use_embedded=on  optimum_pipeline=off  pipeline=on  use_rpm=on  placement_style=Triangular  XmcBlockStatus=1  maskContainerNames=group1  block_type=mult  block_config=sysgen:Mult_config  block_width=598  block_height=876
  Slice Out : Outport
  Valid Out : Outport  Port=2
  wires:
  Pixel 9 X Weight 9/1 -> Combine 8-9/2
  Pixel 7 X Weight 7/1 -> Combine 6-7/2
  Combine (8-9)-(10-11)/1 -> Delay Addition/1
  Combine 10-11/1 -> Combine (8-9)-(10-11)/2
  Pixel 8 X Weight 8/1 -> Combine 8-9/1
  Pixel 10 X Weight 10/1 -> Combine 10-11/1
  Combine (0-1)-(2-3)/1 -> "Combine ((0-1)-(2-3)) - ((4-5)-(6-7)) "/1
  Pixel 1 X Weight 1/1 -> Combine 0-1/2
  Pixel 6 X Weight 6/1 -> Combine 6-7/1
  Combine 6-7/1 -> Combine (4-5)-(6-7)/2
  Combine 4-5/1 -> Combine (4-5)-(6-7)/1
  Combine (4-5)-(6-7)/1 -> "Combine ((0-1)-(2-3)) - ((4-5)-(6-7)) "/2
  Pixel 2 X Weight 2/1 -> Combine 2-3/1
  Pixel 4 X Weight 4/1 -> Combine 4-5/1
  Combine 0-1/1 -> Combine (0-1)-(2-3)/1
  Pixel 5 X Weight 5/1 -> Combine 4-5/2
  Pixel 0 X Weight 0/1 -> Combine 0-1/1
  Pixel 3 X Weight 3/1 -> Combine 2-3/2
  Combine 8-9/1 -> Combine (8-9)-(10-11)/1
  Pixel 11 X Weight 11/1 -> Combine 10-11/2
  Combine 2-3/1 -> Combine (0-1)-(2-3)/2
  Last Combine/1 -> Slice Out/1
  "Combine ((0-1)-(2-3)) - ((4-5)-(6-7)) "/1 -> Last Combine/1
  Delay Addition/1 -> Last Combine/2
  Pixel 0/1 -> Pixel 0 X Weight 0/1
  Weight 0/1 -> Pixel 0 X Weight 0/2
  Pixel 1/1 -> Pixel 1 X Weight 1/1
  Weight 1/1 -> Pixel 1 X Weight 1/2
  Pixel 2/1 -> Pixel 2 X Weight 2/1
  Weight 2/1 -> Pixel 2 X Weight 2/2
  Pixel 3/1 -> Pixel 3 X Weight 3/1
  Weight 3/1 -> Pixel 3 X Weight 3/2
  Pixel 4/1 -> Pixel 4 X Weight 4/1
  Weight 4/1 -> Pixel 4 X Weight 4/2
  Pixel 5/1 -> Pixel 5 X Weight 5/1
  Weight 5/1 -> Pixel 5 X Weight 5/2
  Pixel 6/1 -> Pixel 6 X Weight 6/1
  Weight 6/1 -> Pixel 6 X Weight 6/2
  Pixel 7/1 -> Pixel 7 X Weight 7/1
  Weight 7/1 -> Pixel 7 X Weight 7/2
  Pixel 8/1 -> Pixel 8 X Weight 8/1
  Weight 8/1 -> Pixel 8 X Weight 8/2
  Pixel 9/1 -> Pixel 9 X Weight 9/1
  Weight 9/1 -> Pixel 9 X Weight 9/2
  Pixel 10/1 -> Pixel 10 X Weight 10/1
  Weight 10/1 -> Pixel 10 X Weight 10/2
  Pixel 11/1 -> Pixel 11 X Weight 11/1
  Weight 11/1 -> Pixel 11 X Weight 11/2
  Valid Data/1 -> Delay Addition1/1
  Delay Addition1/1 -> Delay Addition 2/1
  Delay Addition 2/1 -> Delay Addition2/1
  Delay Addition2/1 -> Delay Addition3/1
  Delay Addition3/1 -> Delay Addition4/1
  Delay Addition4/1 -> Valid Out/1
